simulink library "test_1"  (R2022a)
settings: Solver=VariableStepAuto  StartTime=0.0  StopTime=10.0  RelTol=1e-3
settings Model: Creator=q541028  LastModifiedBy=q541028

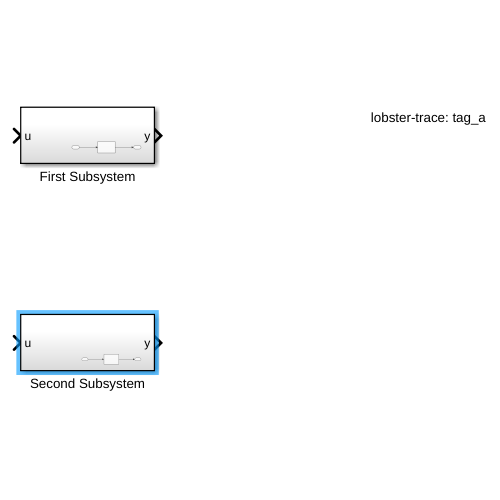
[thumbnail: Simulink's stored preview of the top-level diagram]
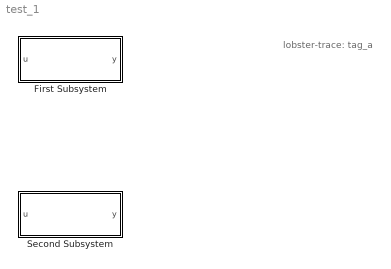
== system test_1 ==
  note: lobster-trace: tag_a
  First Subsystem : Subsystem
  Second Subsystem : Subsystem

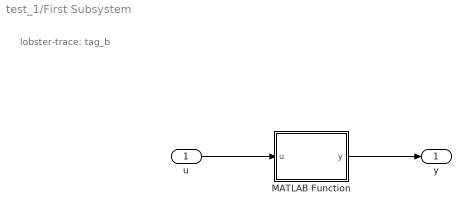
== system test_1/First Subsystem ==
  note: lobster-trace: tag_b
  u : Inport
  MATLAB Function : MATLAB Function  TreatAsAtomicUnit=on
  y : Outport
  wires:
  u/1 -> MATLAB Function/1(u)
  MATLAB Function/1(y) -> y/1

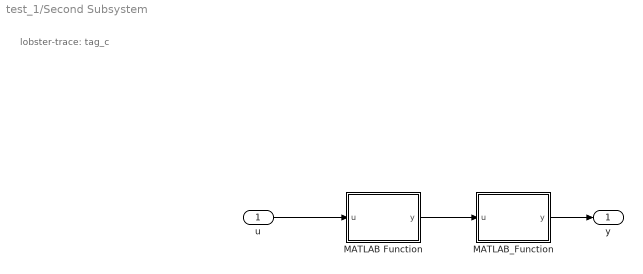
== system test_1/Second Subsystem ==
  note: lobster-trace: tag_c
  u : Inport
  MATLAB Function : MATLAB Function  TreatAsAtomicUnit=on
  MATLAB_Function : MATLAB Function  TreatAsAtomicUnit=on
  y : Outport
  wires:
  u/1 -> MATLAB Function/1(u)
  MATLAB Function/1(y) -> MATLAB_Function/1(u)
  MATLAB_Function/1(y) -> y/1

== matlab function test_1/First Subsystem/MATLAB Function ==
  data: u input; y output
function y = fcn(u)

y = u;

== matlab function test_1/Second Subsystem/MATLAB_Function ==
  data: u input; y output
function y = fcn(u)

y = u;

== matlab function test_1/Second Subsystem/MATLAB Function ==
  data: u input; y output
function y = fcn(u)

y = u;
